simulink library "autolibdatasheetbattery"  (R2019b)
settings: Solver=VariableStepAuto  StartTime=0.0  StopTime=10.0  RelTol=1e-3  EnableMultiTasking=on
libraries: autolibbatterycommon x3
settings Model: ModifiedByFormat=The MathWorks, Inc.  Creator=The MathWorks, Inc.  LastModifiedBy=The MathWorks, Inc.
settings DataIOCC: LimitDataPoints=on  ReturnWorkspaceOutputs=off
settings OptimizationCC: LifeSpan=inf
settings DebuggingCC: AllowSymbolicDim=off  SFUnexpectedBacktrackingDiag=warning  SFNoUnconditionalDefaultTransitionDiag=warning  SFExecutionAtInitializationDiag=none  ArithmeticOperatorsInVariantConditions=warning
settings ModelReferenceCC: PropagateSignalLabelsOutOfModel=off
settings SFSimCC: SimUseLocalCustomCode=off  CustomCodeUndefinedFunction=UseInterfaceOnly
settings RTWCC: RTWUseLocalCustomCode=off
settings CodeAppCC: StateflowObjectComments=on
settings GRTTargetCC: TargetLangStandard=C89/C90 (ANSI)
settings ConfigComp: CovMetricSettings=dw  CovHtmlReporting=on  CovSaveCumulativeToWorkspaceVar=on  CovSaveSingleToWorkspaceVar=on  CovShowResultsExplorer=off  CovExternalEMLEnable=off

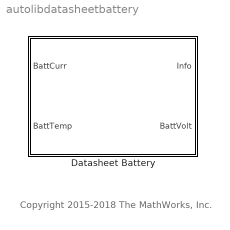
== system autolibdatasheetbattery ==
  note: Copyright 2015-2018 The MathWorks, Inc.
  Datasheet Battery : Subsystem  mask(Datasheet Battery){CapacityCtrl=Parameter, OutputVlt=Unfiltered, BattChargeMax=100, Em=[2.8 3.228 3.284 3.361 3.408 3.427 3.472 3.477 3.493 3.504 3.516 3.528 3.537 3.545 3.555 3.561 3.566 3.576 3.587 3.589 3.594 3.6 3.608 3.61 3.616 3.619 3.626 3.632 3.637 3.64 3.645 3.646 3.652 3.655 3.658 3.661 3.664 3.668 3.673 3.678 3.68 3.681 3.686 3.692 3.699 3.702 3.705 3.71 3.717 3.723 3.728 3.733 3.735 3.742 3.749 3.755 3.761 3.768 3.773 3.78 3.791 3.798 3.798 3.814 3.818 3.825 3.841 3.846 3.855 3.863 3.877 3.885 3.894 3.907 3.919 3.926 3.935 3.944 3.954 3.964 3.974 3.988 3.998 4.014 4.029 4.034 4.047 4.065 4.074 4.086 4.097 4.131 4.126 4.138 4.15 4.18 4.174 4.187 4.207 4.231 4.221], CapLUTBp=[0 0.01 0.02 0.03 0.04 0.05 0.06 0.07 0.08 0.09 0.1 0.11 0.12 0.13 0.14 0.15 0.16 0.17 0.18 0.19 0.2 0.21 0.22 0.23 0.24 0.25 0.26 0.27 0.28 0.29 0.3 0.31 0.32 0.33 0.34 0.35 0.36 0.37 0.38 0.39 0.4 0.41 0.42 0.43 0.44 0.45 0.46 0.47 0.48 0.49 0.5 0.51 0.52 0.53 0.54 0.55 0.56 0.57 0.58 0.59 0.6 0.61 0.62 0.63 0.64 0.65 0.66 0.67 0.68 0.69 0.7 0.71 0.72 0.73 0.74 0.75 0.76 0.77 0.78 0.79 0.8 0.81 0.82 0.83 0.84 0.85 0.86 0.87 0.88 0.89 0.9 0.91 0.92 0.93 0.94 0.95 0.96 0.97 0.98 0.99 1], RInt=[0.008846 0.009319 0.009027 0.00847 0.01032 0.01314;0.006389 0.006554 0.005553 0.005525 0.006043 0.007805;0.004364 0.004101 0.00406 0.003452 0.003846 0.004517;0.002031 0.002563 0.002532 0.00246 0.002716 0.003047;0.001443 0.001825 0.001795 0.001778 0.001924 0.002234;0.0005603 0.0007192 0.0006887 0.0007557 0.0007355 0.001014;0.001028 0.001338 0.001 0.001536 0.001546 0.002789], BattTempBp=[243.1 253.1 263.1 273.1 283.1 298.1 313.1], CapSOCBp=[0 0.2 0.4 0.6 0.8 1], Ns=1, Np=1, BattCapInit=100, Tc=1/1000, Vinit=4.221, RefBlkName='autolibdatasheetbattery/Datasheet Battery'}
      mask prompts: CapacityCtrl "autoblks:autoblkDatasheetBattery:blkPrm_CapacityCtrl"; OutputVlt "autoblks:autoblkDatasheetBattery:blkPrm_OutputVlt"; BattChargeMax "autoblks:autoblkDatasheetBattery:blkPrm_BattChargeMax"; Em "autoblks:autoblkDatasheetBattery:blkPrm_Em"; CapLUTBp "autoblks:autoblkDatasheetBattery:blkPrm_CapLUTBp"; RInt "autoblks:autoblkDatasheetBattery:blkPrm_RInt"; BattTempBp "autoblks:autoblkDatasheetBattery:blkPrm_BattTempBp"; CapSOCBp "autoblks:autoblkDatasheetBattery:blkPrm_CapSOCBp"; Ns "autoblks:autoblkDatasheetBattery:blkPrm_Ns"; Np "autoblks:autoblkDatasheetBattery:blkPrm_Np"; BattCapInit "autoblks:autoblkDatasheetBattery:blkPrm_BattCapInit"; Tc "autoblks:autoblkDatasheetBattery:blkPrm_Tc"; Vinit "autoblks:autoblkDatasheetBattery:blkPrm_Vinit"
      mask help: autoblks:autoblkDatasheetBattery:blkDesc
      mask init:
      | autoicon('autolibdatasheetbattery',gcb,'Initialization');
      mask Help: eval('autoblkshelp(''pbbatterydatasheet'')');
      mask TypeOptions CapacityCtrl: autoblks:autoblkDatasheetBattery:blkCmb_CapacityCtrlExternalInput | autoblks:autoblkDatasheetBattery:blkCmb_CapacityCtrlParameter
      mask TypeOptions OutputVlt: autoblks:autoblkDatasheetBattery:blkCmb_OutputVltFiltered | autoblks:autoblkDatasheetBattery:blkCmb_OutputVltUnfiltered
      mask DialogControl Container3 Prompt: autoblks:autoblkDatasheetBattery:blkDlg_Container3
      mask DialogControl CapacityCtrl Prompt: Initial battery capacity:
      mask DialogControl OutputVlt Prompt: Output battery voltage:
      mask DialogControl ParameterGroupVar Prompt: autoblks:autoblkDatasheetBattery:blkDlg_ParameterGroupVar
      mask DialogControl BattChargeMax Prompt: Rated capacity at nominal temperature, BattChargeMax [Ah]:
      mask DialogControl Em Prompt: Open circuit voltage table data, Em [V]:
      mask DialogControl CapLUTBp Prompt: Open circuit voltage breakpoints 1, CapLUTBp []:
      mask DialogControl RInt Prompt: Internal resistance table data, RInt [Ohms]:
      mask DialogControl BattTempBp Prompt: Battery temperature breakpoints 1, BattTempBp [K]:
      mask DialogControl CapSOCBp Prompt: Battery capacity breakpoints 2, CapSOCBp []:
      mask DialogControl Ns Prompt: Number of cells in series, Ns []:
      mask DialogControl Np Prompt: Number of cells in parallel, Np []:
      mask DialogControl BattCapInit Prompt: Initial battery capacity, BattCapInit [Ah]:
      mask DialogControl Tc Prompt: Output battery voltage time constant, Tc [s]:
      mask DialogControl Vinit Prompt: Output battery voltage initial value, Vinit [V]:
      mask Display:
      | IconInfo = autoicon('autolibdatasheetbattery', gcb, 'DrawCommands');
      | 
      | image(IconInfo.image, IconInfo.position);
      | 
      | for i = 1:numel(IconInfo.lconn)
      |     port_label('lconn', i, IconInfo.lconn{i})
      | end
      | 
      | for j = 1:numel(IconInfo.rconn)
      |     port_label('rconn', j, IconInfo.rconn{j})
      | end
      | 
      | for k = 1:numel(IconInfo.input)
      |     port_label('input', k, IconInfo.input{k})
      | end
      | 
      | for m = 1:numel(IconInfo.output)
      |     port_label('output', m, IconInfo.output{m})
      | end

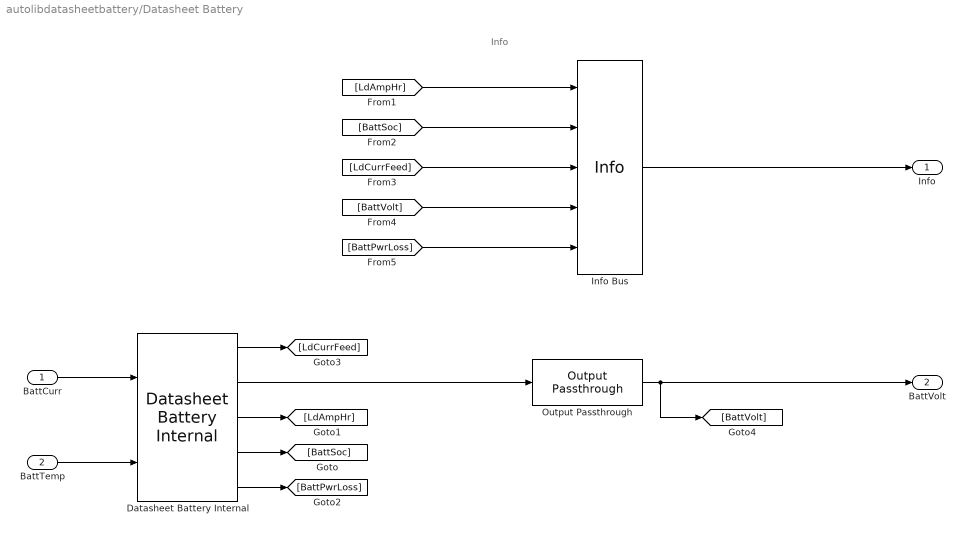
== system autolibdatasheetbattery/Datasheet Battery ==
  note: Info
  BattCurr : Inport  Unit=A
  BattTemp : Inport  Port=2  Unit=K
  Datasheet Battery Internal : autolibbatterycommon/Datasheet Battery Internal  SystemSampleTime=-1  Latency=0  AutoFrameSizeCalculation=off
      settings: SourceProductName=Powertrain Blockset  SourceProductBaseCode=PW
  Info Bus : autolibbatterycommon/Info  RefBlkName='autolibdatasheetbattery/Datasheet Battery'
      settings: SourceProductName=Powertrain Blockset  SourceProductBaseCode=PW
  Output Passthrough : autolibbatterycommon/Output Passthrough  SystemSampleTime=-1  Latency=0  AutoFrameSizeCalculation=off
      settings: SourceProductName=Powertrain Blockset  SourceProductBaseCode=PW
  Info : Outport  VectorParamsAs1DForOutWhenUnconnected=off
  BattVolt : Outport  Port=2  Unit=V  VectorParamsAs1DForOutWhenUnconnected=off
  wires:
  [LdAmpHr] -> Info Bus/1
  [BattSoc] -> Info Bus/2
  Info Bus/1 -> Info/1
  BattCurr/1 -> Datasheet Battery Internal/1
  BattTemp/1 -> Datasheet Battery Internal/2
  Datasheet Battery Internal/4 -> [BattSoc]
  Datasheet Battery Internal/3 -> [LdAmpHr]
  Datasheet Battery Internal/2 -> Output Passthrough/1
  Datasheet Battery Internal/5 -> [BattPwrLoss]
  [LdCurrFeed] -> Info Bus/3
  Datasheet Battery Internal/1 -> [LdCurrFeed]
  [BattVolt] -> Info Bus/4
  Output Passthrough/1 -> [BattVolt], BattVolt/1
  [BattPwrLoss] -> Info Bus/5
